simulink model "RC_Logitech"  (R2017b)
settings: Solver=FixedStepDiscrete  StartTime=0.0  StopTime=inf  FixedStep=0.02  RelTol=1e-3
libraries: simulink x16, aerolibanimutils x1
settings Model: Creator=juju  LastModifiedBy=zht
settings DataIOCC: LimitDataPoints=on  SaveFormat=Array  SaveOutput=off
settings OptimizationCC: BlockReduction=off  BooleanDataType=off  LifeSpan=inf
settings DebuggingCC: ConsistencyChecking=error  SignalInfNanChecking=error  SignalRangeChecking=error  ReadBeforeWriteMsg=EnableAllAsError  WriteAfterWriteMsg=EnableAllAsError  WriteAfterReadMsg=EnableAllAsError  AlgebraicLoopMsg=error  ArtificialAlgebraicLoopMsg=error  SaveWithDisabledLinksMsg=error  SaveWithParameterizedLinksMsg=error  BlockPriorityViolationMsg=error  MinStepSizeMsg=error  TimeAdjustmentMsg=warning  SolverPrmCheckMsg=error  InheritedTsInSrcMsg=error  SingleTaskRateTransMsg=error  TasksWithSamePriorityMsg=error  SigSpecEnsureSampleTimeMsg=error  CheckMatrixSingularityMsg=error  IntegerOverflowMsg=error  ParameterUnderflowMsg=error  ParameterPrecisionLossMsg=error  ParameterTunabilityLossMsg=error  FixptConstUnderflowMsg=error  FixptConstOverflowMsg=error  FixptConstPrecisionLossMsg=error  UnderSpecifiedDataTypeMsg=warning  UnnecessaryDatatypeConvMsg=warning  VectorMatrixConversionMsg=error  SignalLabelMismatchMsg=error  UnconnectedInputMsg=error  UnconnectedOutputMsg=error  UnconnectedLineMsg=error  SFcnCompatibilityMsg=error  UniqueDataStoreMsg=error  BusObjectLabelMismatch=error  RootOutportRequireBusObject=error  ModelReferenceIOMsg=error  ModelReferenceVersionMismatchMessage=error  ModelReferenceIOMismatchMessage=error  UnknownTsInhSupMsg=error  ModelReferenceDataLoggingMessage=error  StateNameClashWarn=warning  SimStateInterfaceChecksumMismatchMsg=error  StrictBusMsg=ErrorOnBusTreatedAsVector  BusNameAdapt=ErrorWithoutRepair  NonBusSignalsTreatedAsBus=error  SFUnusedDataAndEventsDiag=error  SFInvalidInputDataAccessInChartInitDiag=error  SFTransitionOutsideNaturalParentDiag=error  SFUnreachableExecutionPathDiag=error  SFUndirectedBroadcastEventsDiag=error  SFTransitionActionBeforeConditionDiag=error  SFTemporalDelaySmallerThanSampleTimeDiag=error  SFSelfTransitionDiag=error  SFExecutionAtInitializationDiag=error  SFMachineParentedDataDiag=error  IntegerSaturationMsg=error
settings HardwareCC: ProdBitPerPointer=32  ProdBitPerSizeT=32  ProdBitPerPtrDiffT=32  ProdLargestAtomicFloat=None  ProdIntDivRoundTo=Undefined  ProdEndianess=Unspecified  ProdWordSize=32  ProdHWDeviceType=32-bit Generic  TargetBitPerLong=64  TargetBitPerPointer=64  TargetBitPerSizeT=64  TargetBitPerPtrDiffT=64  TargetLongLongMode=on  TargetIntDivRoundTo=Zero  TargetEndianess=LittleEndian  TargetWordSize=64  TargetHWDeviceType=MATLAB Host  ProdEqTarget=off
settings ModelReferenceCC: PropagateSignalLabelsOutOfModel=off
settings CodeAppCC: StateflowObjectComments=on
settings GRTTargetCC: TargetLangStandard=C89/C90 (ANSI)  GeneratePreprocessorConditionals=Disable all
settings ConfigComp: CovMetricSettings=dw  CovHtmlReporting=on  CovSaveCumulativeToWorkspaceVar=on  CovSaveSingleToWorkspaceVar=on  CovExternalEMLEnable=off  CovSFcnEnable=off
settings SimscapeCC: SimscapeNormalizeSystem=off

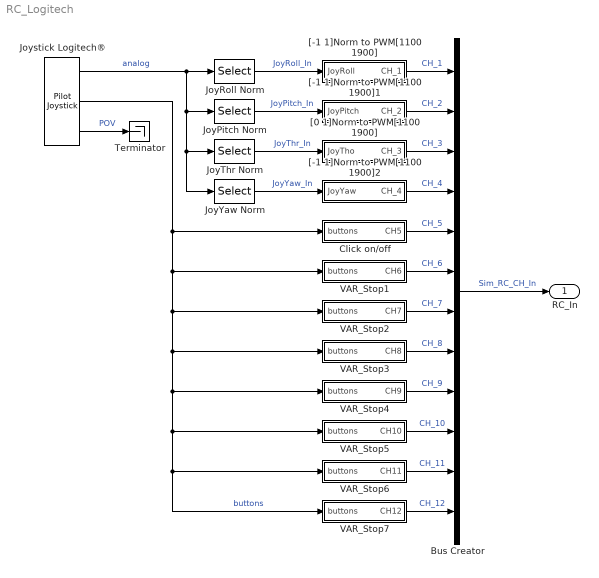
== system RC_Logitech ==
  Bus Creator : BusCreator  Inputs=12  OutDataTypeStr=Bus: RC_In_BUS  NonVirtualBus=on
  Click on/off : Subsystem
  JoyPitch Norm : Selector  InputPortWidth=6  IndexOptions=Index vector (dialog)  Indices=[2]  OutputSizes=1
  JoyRoll Norm : Selector  InputPortWidth=6  IndexOptions=Index vector (dialog)  Indices=[1]  OutputSizes=1
  JoyThr Norm : Selector  InputPortWidth=6  IndexOptions=Index vector (dialog)  Indices=[3]  OutputSizes=1
  JoyYaw Norm : Selector  InputPortWidth=6  IndexOptions=Index vector (dialog)  Indices=[4]  OutputSizes=1
  Joystick Logitech® : aerolibanimutils/Pilot Joystick  JoystickID=None  OutputConfiguration=AllOutputs  SampleTime=0.02
  Terminator : Terminator
  VAR_Stop1 : Subsystem
  VAR_Stop2 : Subsystem
  VAR_Stop3 : Subsystem
  VAR_Stop4 : Subsystem
  VAR_Stop5 : Subsystem
  VAR_Stop6 : Subsystem
  VAR_Stop7 : Subsystem
  "[-1 1]Norm to PWM[1100 1900]" : Subsystem
  "[-1 1]Norm to PWM[1100 1900]1" : Subsystem
  "[-1 1]Norm to PWM[1100 1900]2" : Subsystem
  "[0 1]Norm to PWM[1100 1900]" : Subsystem
  RC_In : Outport  OutDataTypeStr=Bus: RC_In_BUS
  wires:
  Joystick Logitech®/2 -> Click on/off/1(buttons), VAR_Stop1/1(buttons), VAR_Stop2/1(buttons), VAR_Stop3/1(buttons), VAR_Stop4/1(buttons), VAR_Stop5/1(buttons), VAR_Stop6/1(buttons), VAR_Stop7/1(buttons)  "buttons"
  Joystick Logitech®/3 -> Terminator/1  "POV"
  "[-1 1]Norm to PWM[1100 1900]"/1(CH_1) -> Bus Creator/1  "CH_1"
  "[-1 1]Norm to PWM[1100 1900]1"/1(CH_2) -> Bus Creator/2  "CH_2"
  "[0 1]Norm to PWM[1100 1900]"/1(CH_3) -> Bus Creator/3  "CH_3"
  "[-1 1]Norm to PWM[1100 1900]2"/1(CH_4) -> Bus Creator/4  "CH_4"
  Click on/off/1(CH5) -> Bus Creator/5  "CH_5"
  VAR_Stop1/1(CH6) -> Bus Creator/6  "CH_6"
  VAR_Stop2/1(CH7) -> Bus Creator/7  "CH_7"
  VAR_Stop3/1(CH8) -> Bus Creator/8  "CH_8"
  VAR_Stop5/1(CH10) -> Bus Creator/10  "CH_10"
  VAR_Stop4/1(CH9) -> Bus Creator/9  "CH_9"
  VAR_Stop6/1(CH11) -> Bus Creator/11  "CH_11"
  VAR_Stop7/1(CH12) -> Bus Creator/12  "CH_12"
  Joystick Logitech®/1 -> JoyYaw Norm/1, JoyThr Norm/1, JoyPitch Norm/1, JoyRoll Norm/1  "analog"
  JoyRoll Norm/1 -> "[-1 1]Norm to PWM[1100 1900]"/1(JoyRoll)  "JoyRoll_In"
  JoyPitch Norm/1 -> "[-1 1]Norm to PWM[1100 1900]1"/1(JoyPitch)  "JoyPitch_In"
  JoyThr Norm/1 -> "[0 1]Norm to PWM[1100 1900]"/1(JoyTho)  "JoyThr_In"
  JoyYaw Norm/1 -> "[-1 1]Norm to PWM[1100 1900]2"/1(JoyYaw)  "JoyYaw_In"
  Bus Creator/1 -> RC_In/1  "Sim_RC_CH_In"

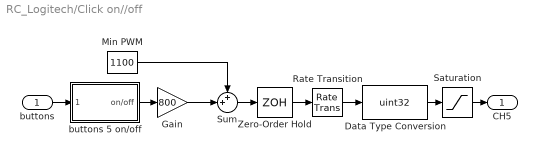
== system RC_Logitech/Click on//off ==
  buttons : Inport
  Data Type Conversion : DataTypeConversion  OutDataTypeStr=uint32
  Gain : Gain  Gain=800
  Min PWM : Constant  Value=1100
  Rate Transition : RateTransition
  Saturation : Saturate  UpperLimit=1900  LowerLimit=1100
  Sum : Sum  Inputs=++|
  Zero-Order Hold : ZeroOrderHold  SampleTime=0.02
  buttons 5 on/off : Subsystem
  CH5 : Outport
  wires:
  buttons/1 -> buttons 5 on/off/1(buttons)
  Min PWM/1 -> Sum/1
  Rate Transition/1 -> Data Type Conversion/1
  buttons 5 on/off/1(on/off) -> Gain/1
  Gain/1 -> Sum/2
  Data Type Conversion/1 -> Saturation/1
  Sum/1 -> Zero-Order Hold/1
  Zero-Order Hold/1 -> Rate Transition/1
  Saturation/1 -> CH5/1

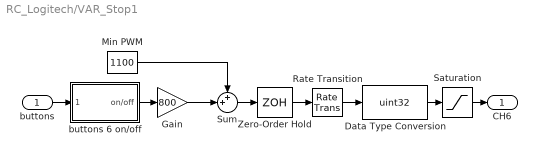
== system RC_Logitech/VAR_Stop1 ==
  buttons : Inport
  Data Type Conversion : DataTypeConversion  OutDataTypeStr=uint32
  Gain : Gain  Gain=800
  Min PWM : Constant  Value=1100
  Rate Transition : RateTransition
  Saturation : Saturate  UpperLimit=1900  LowerLimit=1100
  Sum : Sum  Inputs=++|
  Zero-Order Hold : ZeroOrderHold  SampleTime=0.02
  buttons 6 on/off : Subsystem
  CH6 : Outport
  wires:
  Saturation/1 -> CH6/1
  Zero-Order Hold/1 -> Rate Transition/1
  Sum/1 -> Zero-Order Hold/1
  Data Type Conversion/1 -> Saturation/1
  Gain/1 -> Sum/2
  buttons 6 on/off/1(on/off) -> Gain/1
  Rate Transition/1 -> Data Type Conversion/1
  Min PWM/1 -> Sum/1
  buttons/1 -> buttons 6 on/off/1(buttons)

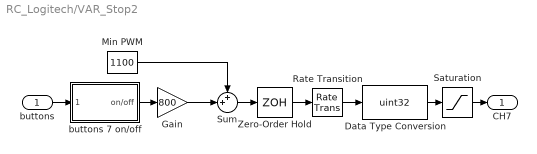
== system RC_Logitech/VAR_Stop2 ==
  buttons : Inport
  Data Type Conversion : DataTypeConversion  OutDataTypeStr=uint32
  Gain : Gain  Gain=800
  Min PWM : Constant  Value=1100
  Rate Transition : RateTransition
  Saturation : Saturate  UpperLimit=1900  LowerLimit=1100
  Sum : Sum  Inputs=++|
  Zero-Order Hold : ZeroOrderHold  SampleTime=0.02
  buttons 7 on/off : Subsystem
  CH7 : Outport
  wires:
  buttons/1 -> buttons 7 on/off/1(buttons)
  Min PWM/1 -> Sum/1
  Rate Transition/1 -> Data Type Conversion/1
  buttons 7 on/off/1(on/off) -> Gain/1
  Gain/1 -> Sum/2
  Data Type Conversion/1 -> Saturation/1
  Sum/1 -> Zero-Order Hold/1
  Zero-Order Hold/1 -> Rate Transition/1
  Saturation/1 -> CH7/1

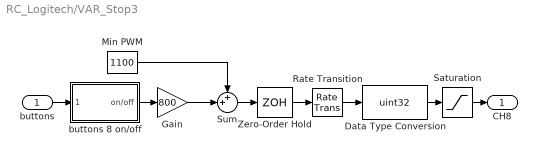
== system RC_Logitech/VAR_Stop3 ==
  buttons : Inport
  Data Type Conversion : DataTypeConversion  OutDataTypeStr=uint32
  Gain : Gain  Gain=800
  Min PWM : Constant  Value=1100
  Rate Transition : RateTransition
  Saturation : Saturate  UpperLimit=1900  LowerLimit=1100
  Sum : Sum  Inputs=++|
  Zero-Order Hold : ZeroOrderHold  SampleTime=0.02
  buttons 8 on/off : Subsystem
  CH8 : Outport
  wires:
  Saturation/1 -> CH8/1
  Zero-Order Hold/1 -> Rate Transition/1
  Sum/1 -> Zero-Order Hold/1
  Data Type Conversion/1 -> Saturation/1
  Gain/1 -> Sum/2
  buttons 8 on/off/1(on/off) -> Gain/1
  Rate Transition/1 -> Data Type Conversion/1
  Min PWM/1 -> Sum/1
  buttons/1 -> buttons 8 on/off/1(buttons)

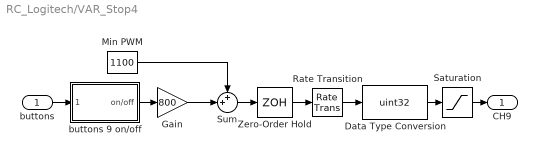
== system RC_Logitech/VAR_Stop4 ==
  buttons : Inport
  Data Type Conversion : DataTypeConversion  OutDataTypeStr=uint32
  Gain : Gain  Gain=800
  Min PWM : Constant  Value=1100
  Rate Transition : RateTransition
  Saturation : Saturate  UpperLimit=1900  LowerLimit=1100
  Sum : Sum  Inputs=++|
  Zero-Order Hold : ZeroOrderHold  SampleTime=0.02
  buttons 9 on/off : Subsystem
  CH9 : Outport
  wires:
  buttons/1 -> buttons 9 on/off/1(buttons)
  Min PWM/1 -> Sum/1
  Rate Transition/1 -> Data Type Conversion/1
  buttons 9 on/off/1(on/off) -> Gain/1
  Gain/1 -> Sum/2
  Data Type Conversion/1 -> Saturation/1
  Sum/1 -> Zero-Order Hold/1
  Zero-Order Hold/1 -> Rate Transition/1
  Saturation/1 -> CH9/1

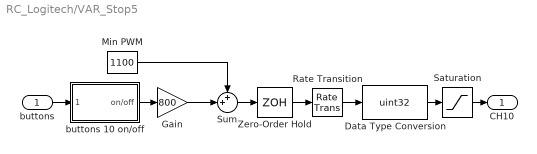
== system RC_Logitech/VAR_Stop5 ==
  buttons : Inport
  Data Type Conversion : DataTypeConversion  OutDataTypeStr=uint32
  Gain : Gain  Gain=800
  Min PWM : Constant  Value=1100
  Rate Transition : RateTransition
  Saturation : Saturate  UpperLimit=1900  LowerLimit=1100
  Sum : Sum  Inputs=++|
  Zero-Order Hold : ZeroOrderHold  SampleTime=0.02
  buttons 10 on/off : Subsystem
  CH10 : Outport
  wires:
  Saturation/1 -> CH10/1
  Zero-Order Hold/1 -> Rate Transition/1
  Sum/1 -> Zero-Order Hold/1
  Data Type Conversion/1 -> Saturation/1
  Gain/1 -> Sum/2
  buttons 10 on/off/1(on/off) -> Gain/1
  Rate Transition/1 -> Data Type Conversion/1
  Min PWM/1 -> Sum/1
  buttons/1 -> buttons 10 on/off/1(buttons)

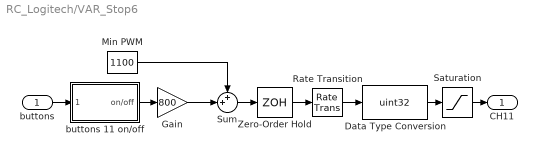
== system RC_Logitech/VAR_Stop6 ==
  buttons : Inport
  Data Type Conversion : DataTypeConversion  OutDataTypeStr=uint32
  Gain : Gain  Gain=800
  Min PWM : Constant  Value=1100
  Rate Transition : RateTransition
  Saturation : Saturate  UpperLimit=1900  LowerLimit=1100
  Sum : Sum  Inputs=++|
  Zero-Order Hold : ZeroOrderHold  SampleTime=0.02
  buttons 11 on/off : Subsystem
  CH11 : Outport
  wires:
  buttons/1 -> buttons 11 on/off/1(buttons)
  Min PWM/1 -> Sum/1
  Rate Transition/1 -> Data Type Conversion/1
  buttons 11 on/off/1(on/off) -> Gain/1
  Gain/1 -> Sum/2
  Data Type Conversion/1 -> Saturation/1
  Sum/1 -> Zero-Order Hold/1
  Zero-Order Hold/1 -> Rate Transition/1
  Saturation/1 -> CH11/1

== system RC_Logitech/VAR_Stop7 ==
  buttons : Inport
  Data Type Conversion : DataTypeConversion  OutDataTypeStr=uint32
  Gain : Gain  Gain=800
  Min PWM : Constant  Value=1100
  Rate Transition : RateTransition
  Saturation : Saturate  UpperLimit=1900  LowerLimit=1100
  Sum : Sum  Inputs=++|
  Zero-Order Hold : ZeroOrderHold  SampleTime=0.02
  buttons 12 on/off : Subsystem
  CH12 : Outport
  wires:
  Saturation/1 -> CH12/1
  Zero-Order Hold/1 -> Rate Transition/1
  Sum/1 -> Zero-Order Hold/1
  Data Type Conversion/1 -> Saturation/1
  Gain/1 -> Sum/2
  buttons 12 on/off/1(on/off) -> Gain/1
  Rate Transition/1 -> Data Type Conversion/1
  Min PWM/1 -> Sum/1
  buttons/1 -> buttons 12 on/off/1(buttons)

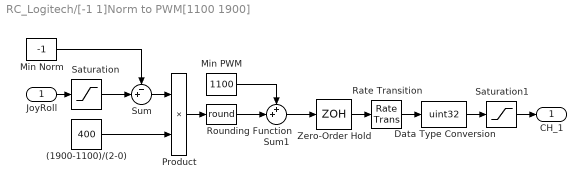
== system RC_Logitech/[-1 1]Norm to PWM[1100 1900] ==
  JoyRoll : Inport  OutDataTypeStr=double  Unit=1  PortDimensions=1
  (1900-1100)/(2-0) : Constant  Value=400  OutDataTypeStr=uint32
  Data Type Conversion : DataTypeConversion  OutDataTypeStr=uint32
  Min Norm : Constant  Value=-1
  Min PWM : Constant  Value=1100  OutDataTypeStr=uint32
  Product : Product  Inputs=**
  Rate Transition : RateTransition
  Rounding Function : Rounding  Operator=round
  Saturation : Saturate  UpperLimit=1  LowerLimit=-1
  Saturation1 : Saturate  UpperLimit=1900  LowerLimit=1100
  Sum : Sum  Inputs=-+|
  Sum1 : Sum  Inputs=++|
  Zero-Order Hold : ZeroOrderHold  SampleTime=0.02
  CH_1 : Outport  OutMin=[1100]  OutMax=[1900]  OutDataTypeStr=uint32  PortDimensions=1
  wires:
  JoyRoll/1 -> Saturation/1
  Saturation/1 -> Sum/2
  Min Norm/1 -> Sum/1
  Sum/1 -> Product/1
  (1900-1100)/(2-0)/1 -> Product/2
  Product/1 -> Rounding Function/1
  Min PWM/1 -> Sum1/1
  Sum1/1 -> Zero-Order Hold/1
  Rounding Function/1 -> Sum1/2
  Data Type Conversion/1 -> Saturation1/1
  Zero-Order Hold/1 -> Rate Transition/1
  Rate Transition/1 -> Data Type Conversion/1
  Saturation1/1 -> CH_1/1

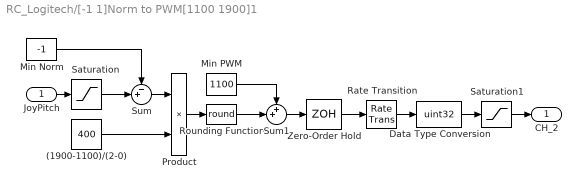
== system RC_Logitech/[-1 1]Norm to PWM[1100 1900]1 ==
  JoyPitch : Inport  OutDataTypeStr=double  Unit=1  PortDimensions=1
  (1900-1100)/(2-0) : Constant  Value=400
  Data Type Conversion : DataTypeConversion  OutDataTypeStr=uint32
  Min Norm : Constant  Value=-1
  Min PWM : Constant  Value=1100
  Product : Product  Inputs=**
  Rate Transition : RateTransition
  Rounding Function : Rounding  Operator=round
  Saturation : Saturate  UpperLimit=1  LowerLimit=-1
  Saturation1 : Saturate  UpperLimit=1900  LowerLimit=1100
  Sum : Sum  Inputs=-+|
  Sum1 : Sum  Inputs=++|
  Zero-Order Hold : ZeroOrderHold  SampleTime=0.02
  CH_2 : Outport  OutMin=[1100]  OutMax=[1900]  OutDataTypeStr=uint32  PortDimensions=1
  wires:
  Data Type Conversion/1 -> Saturation1/1
  Rounding Function/1 -> Sum1/2
  Min PWM/1 -> Sum1/1
  Product/1 -> Rounding Function/1
  (1900-1100)/(2-0)/1 -> Product/2
  Sum/1 -> Product/1
  Min Norm/1 -> Sum/1
  Saturation/1 -> Sum/2
  JoyPitch/1 -> Saturation/1
  Zero-Order Hold/1 -> Rate Transition/1
  Rate Transition/1 -> Data Type Conversion/1
  Saturation1/1 -> CH_2/1
  Sum1/1 -> Zero-Order Hold/1

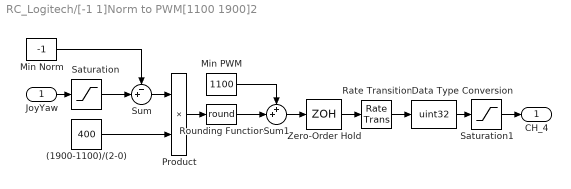
== system RC_Logitech/[-1 1]Norm to PWM[1100 1900]2 ==
  JoyYaw : Inport  OutDataTypeStr=double  Unit=1  PortDimensions=1
  (1900-1100)/(2-0) : Constant  Value=400
  Data Type Conversion : DataTypeConversion  OutDataTypeStr=uint32
  Min Norm : Constant  Value=-1
  Min PWM : Constant  Value=1100
  Product : Product  Inputs=**
  Rate Transition : RateTransition
  Rounding Function : Rounding  Operator=round
  Saturation : Saturate  UpperLimit=1  LowerLimit=-1
  Saturation1 : Saturate  UpperLimit=1900  LowerLimit=1100
  Sum : Sum  Inputs=-+|
  Sum1 : Sum  Inputs=++|
  Zero-Order Hold : ZeroOrderHold  SampleTime=0.02
  CH_4 : Outport  OutMin=[1100]  OutMax=[1900]  OutDataTypeStr=uint32  PortDimensions=1
  wires:
  JoyYaw/1 -> Saturation/1
  Saturation/1 -> Sum/2
  Min Norm/1 -> Sum/1
  Sum/1 -> Product/1
  (1900-1100)/(2-0)/1 -> Product/2
  Product/1 -> Rounding Function/1
  Min PWM/1 -> Sum1/1
  Sum1/1 -> Zero-Order Hold/1
  Rounding Function/1 -> Sum1/2
  Zero-Order Hold/1 -> Rate Transition/1
  Rate Transition/1 -> Data Type Conversion/1
  Data Type Conversion/1 -> Saturation1/1
  Saturation1/1 -> CH_4/1

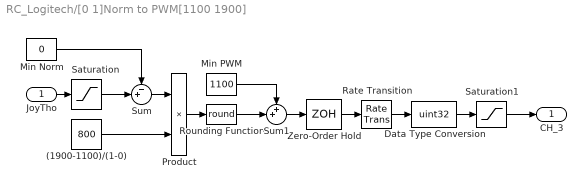
== system RC_Logitech/[0 1]Norm to PWM[1100 1900] ==
  JoyTho : Inport  OutDataTypeStr=double  Unit=1  PortDimensions=1
  (1900-1100)/(1-0) : Constant  Value=800
  Data Type Conversion : DataTypeConversion  OutDataTypeStr=uint32
  Min Norm : Constant  Value=0
  Min PWM : Constant  Value=1100
  Product : Product  Inputs=**
  Rate Transition : RateTransition
  Rounding Function : Rounding  Operator=round
  Saturation : Saturate  UpperLimit=1  LowerLimit=-1
  Saturation1 : Saturate  UpperLimit=1900  LowerLimit=1100
  Sum : Sum  Inputs=-+|
  Sum1 : Sum  Inputs=++|
  Zero-Order Hold : ZeroOrderHold  SampleTime=0.02
  CH_3 : Outport  OutMin=[1100]  OutMax=[1900]  OutDataTypeStr=uint32  PortDimensions=1
  wires:
  JoyTho/1 -> Saturation/1
  Saturation/1 -> Sum/2
  Min Norm/1 -> Sum/1
  Sum/1 -> Product/1
  (1900-1100)/(1-0)/1 -> Product/2
  Product/1 -> Rounding Function/1
  Min PWM/1 -> Sum1/1
  Rounding Function/1 -> Sum1/2
  Zero-Order Hold/1 -> Rate Transition/1
  Rate Transition/1 -> Data Type Conversion/1
  Data Type Conversion/1 -> Saturation1/1
  Sum1/1 -> Zero-Order Hold/1
  Saturation1/1 -> CH_3/1

== system RC_Logitech/Click on//off/buttons 5 on//off ==
  buttons : Inport
  ButtonOnOff : MATLAB Function  TreatAsAtomicUnit=on
  Compare To Constant : simulink/Logic and Bit Operations/Compare To Constant  relop===  const=1  OutDataTypeStr=boolean
  Data Type Conversion3 : DataTypeConversion  OutDataTypeStr=double
  Joystick button 5 : simulink/Logic and Bit Operations/Compare To Constant  relop===  const=16  OutDataTypeStr=boolean
  bts : Subsystem  TreatAsAtomicUnit=on
  on/off : Outport  OutDataTypeStr=boolean  PortDimensions=1
  wires:
  Data Type Conversion3/1 -> ButtonOnOff/1(bts)
  Compare To Constant/1 -> on/off/1
  Joystick button 5/1 -> bts/1(In1)
  buttons/1 -> Joystick button 5/1, bts/Trigger
  bts/1(Out1) -> Data Type Conversion3/1
  ButtonOnOff/1(led) -> Compare To Constant/1

== system RC_Logitech/VAR_Stop1/buttons 6 on//off ==
  buttons : Inport
  ButtonOnOff : MATLAB Function  TreatAsAtomicUnit=on
  Compare To Constant : simulink/Logic and Bit Operations/Compare To Constant  relop===  const=1  OutDataTypeStr=boolean
  Data Type Conversion3 : DataTypeConversion  OutDataTypeStr=double
  Joystick button : simulink/Logic and Bit Operations/Compare To Constant  relop===  const=32  OutDataTypeStr=boolean
  bts : Subsystem  TreatAsAtomicUnit=on
  on/off : Outport  OutDataTypeStr=boolean  PortDimensions=1
  wires:
  ButtonOnOff/1(led) -> Compare To Constant/1
  bts/1(Out1) -> Data Type Conversion3/1
  buttons/1 -> bts/Trigger, Joystick button/1
  Joystick button/1 -> bts/1(In1)
  Compare To Constant/1 -> on/off/1
  Data Type Conversion3/1 -> ButtonOnOff/1(bts)

== system RC_Logitech/VAR_Stop2/buttons 7 on//off ==
  buttons : Inport
  ButtonOnOff : MATLAB Function  TreatAsAtomicUnit=on
  Compare To Constant : simulink/Logic and Bit Operations/Compare To Constant  relop===  const=1  OutDataTypeStr=boolean
  Data Type Conversion3 : DataTypeConversion  OutDataTypeStr=double
  Joystick button : simulink/Logic and Bit Operations/Compare To Constant  relop===  const=64  OutDataTypeStr=boolean
  bts : Subsystem  TreatAsAtomicUnit=on
  on/off : Outport  OutDataTypeStr=boolean  PortDimensions=1
  wires:
  Data Type Conversion3/1 -> ButtonOnOff/1(bts)
  Compare To Constant/1 -> on/off/1
  Joystick button/1 -> bts/1(In1)
  buttons/1 -> Joystick button/1, bts/Trigger
  bts/1(Out1) -> Data Type Conversion3/1
  ButtonOnOff/1(led) -> Compare To Constant/1

== system RC_Logitech/VAR_Stop3/buttons 8 on//off ==
  buttons : Inport
  ButtonOnOff : MATLAB Function  TreatAsAtomicUnit=on
  Compare To Constant : simulink/Logic and Bit Operations/Compare To Constant  relop===  const=1  OutDataTypeStr=boolean
  Data Type Conversion3 : DataTypeConversion  OutDataTypeStr=double
  Joystick button : simulink/Logic and Bit Operations/Compare To Constant  relop===  const=128  OutDataTypeStr=boolean
  bts : Subsystem  TreatAsAtomicUnit=on
  on/off : Outport  OutDataTypeStr=boolean  PortDimensions=1
  wires:
  ButtonOnOff/1(led) -> Compare To Constant/1
  bts/1(Out1) -> Data Type Conversion3/1
  buttons/1 -> bts/Trigger, Joystick button/1
  Joystick button/1 -> bts/1(In1)
  Compare To Constant/1 -> on/off/1
  Data Type Conversion3/1 -> ButtonOnOff/1(bts)

== system RC_Logitech/VAR_Stop4/buttons 9 on//off ==
  buttons : Inport
  ButtonOnOff : MATLAB Function  TreatAsAtomicUnit=on
  Compare To Constant : simulink/Logic and Bit Operations/Compare To Constant  relop===  const=1  OutDataTypeStr=boolean
  Data Type Conversion3 : DataTypeConversion  OutDataTypeStr=double
  Joystick button : simulink/Logic and Bit Operations/Compare To Constant  relop===  const=256  OutDataTypeStr=boolean
  bts : Subsystem  TreatAsAtomicUnit=on
  on/off : Outport  OutDataTypeStr=boolean  PortDimensions=1
  wires:
  Data Type Conversion3/1 -> ButtonOnOff/1(bts)
  Compare To Constant/1 -> on/off/1
  Joystick button/1 -> bts/1(In1)
  buttons/1 -> Joystick button/1, bts/Trigger
  bts/1(Out1) -> Data Type Conversion3/1
  ButtonOnOff/1(led) -> Compare To Constant/1

== system RC_Logitech/VAR_Stop5/buttons 10 on//off ==
  buttons : Inport
  ButtonOnOff : MATLAB Function  TreatAsAtomicUnit=on
  Compare To Constant : simulink/Logic and Bit Operations/Compare To Constant  relop===  const=1  OutDataTypeStr=boolean
  Data Type Conversion3 : DataTypeConversion  OutDataTypeStr=double
  Joystick button : simulink/Logic and Bit Operations/Compare To Constant  relop===  const=512  OutDataTypeStr=boolean
  bts : Subsystem  TreatAsAtomicUnit=on
  on/off : Outport  OutDataTypeStr=boolean  PortDimensions=1
  wires:
  ButtonOnOff/1(led) -> Compare To Constant/1
  bts/1(Out1) -> Data Type Conversion3/1
  buttons/1 -> bts/Trigger, Joystick button/1
  Joystick button/1 -> bts/1(In1)
  Compare To Constant/1 -> on/off/1
  Data Type Conversion3/1 -> ButtonOnOff/1(bts)

== system RC_Logitech/VAR_Stop6/buttons 11 on//off ==
  buttons : Inport
  ButtonOnOff : MATLAB Function  TreatAsAtomicUnit=on
  Compare To Constant : simulink/Logic and Bit Operations/Compare To Constant  relop===  const=1  OutDataTypeStr=boolean
  Data Type Conversion3 : DataTypeConversion  OutDataTypeStr=double
  Joystick button : simulink/Logic and Bit Operations/Compare To Constant  relop===  const=1024  OutDataTypeStr=boolean
  bts : Subsystem  TreatAsAtomicUnit=on
  on/off : Outport  OutDataTypeStr=boolean  PortDimensions=1
  wires:
  Data Type Conversion3/1 -> ButtonOnOff/1(bts)
  Compare To Constant/1 -> on/off/1
  Joystick button/1 -> bts/1(In1)
  buttons/1 -> Joystick button/1, bts/Trigger
  bts/1(Out1) -> Data Type Conversion3/1
  ButtonOnOff/1(led) -> Compare To Constant/1

== system RC_Logitech/VAR_Stop7/buttons 12 on//off ==
  buttons : Inport
  ButtonOnOff : MATLAB Function  TreatAsAtomicUnit=on
  Compare To Constant : simulink/Logic and Bit Operations/Compare To Constant  relop===  const=1  OutDataTypeStr=boolean
  Data Type Conversion3 : DataTypeConversion  OutDataTypeStr=double
  Joystick button : simulink/Logic and Bit Operations/Compare To Constant  relop===  const=2048  OutDataTypeStr=boolean
  bts : Subsystem  TreatAsAtomicUnit=on
  on/off : Outport  OutDataTypeStr=boolean  PortDimensions=1
  wires:
  ButtonOnOff/1(led) -> Compare To Constant/1
  bts/1(Out1) -> Data Type Conversion3/1
  buttons/1 -> bts/Trigger, Joystick button/1
  Joystick button/1 -> bts/1(In1)
  Compare To Constant/1 -> on/off/1
  Data Type Conversion3/1 -> ButtonOnOff/1(bts)

== system RC_Logitech/Click on//off/buttons 5 on//off/bts ==
  In1 : Inport
  Trigger : TriggerPort  TriggerType=either  VariantControl=Variant  InitialTriggerSignalState=positive
  Out1 : Outport
  wires:
  In1/1 -> Out1/1

== system RC_Logitech/VAR_Stop1/buttons 6 on//off/bts ==
  In1 : Inport
  Trigger : TriggerPort  TriggerType=either  VariantControl=Variant  InitialTriggerSignalState=positive
  Out1 : Outport
  wires:
  In1/1 -> Out1/1

== system RC_Logitech/VAR_Stop2/buttons 7 on//off/bts ==
  In1 : Inport
  Trigger : TriggerPort  TriggerType=either  VariantControl=Variant  InitialTriggerSignalState=positive
  Out1 : Outport
  wires:
  In1/1 -> Out1/1

== system RC_Logitech/VAR_Stop3/buttons 8 on//off/bts ==
  In1 : Inport
  Trigger : TriggerPort  TriggerType=either  VariantControl=Variant  InitialTriggerSignalState=positive
  Out1 : Outport
  wires:
  In1/1 -> Out1/1

== system RC_Logitech/VAR_Stop4/buttons 9 on//off/bts ==
  In1 : Inport
  Trigger : TriggerPort  TriggerType=either  VariantControl=Variant  InitialTriggerSignalState=positive
  Out1 : Outport
  wires:
  In1/1 -> Out1/1

== system RC_Logitech/VAR_Stop5/buttons 10 on//off/bts ==
  In1 : Inport
  Trigger : TriggerPort  TriggerType=either  VariantControl=Variant  InitialTriggerSignalState=positive
  Out1 : Outport
  wires:
  In1/1 -> Out1/1

== system RC_Logitech/VAR_Stop6/buttons 11 on//off/bts ==
  In1 : Inport
  Trigger : TriggerPort  TriggerType=either  VariantControl=Variant  InitialTriggerSignalState=positive
  Out1 : Outport
  wires:
  In1/1 -> Out1/1

== system RC_Logitech/VAR_Stop7/buttons 12 on//off/bts ==
  In1 : Inport
  Trigger : TriggerPort  TriggerType=either  VariantControl=Variant  InitialTriggerSignalState=positive
  Out1 : Outport
  wires:
  In1/1 -> Out1/1

== matlab function RC_Logitech/VAR_Stop1/buttons 6 on//off/ButtonOnOff ==
  data: bts input; led output
function led = ButtonOnOff(bts)

persistent btsb                                                            % Initialization(To initialize a variable in embedded function) 
if isempty(btsb)
    btsb = 0;
end

persistent leds
if isempty(leds)
    leds = 0;
end

if ((bts~=btsb) && (bts ==1))                                              % bts is the button on or off in this time step 
    if (leds == 0)
        leds = 1;
    else
        leds = 0;
    end
    btsb = bts;                                                            % btsb is the button on or of in before time step    
end

if ((bts~=btsb) && (bts ==0))
    btsb = bts;
end
led = leds;                                                                % led on or off
%  end

== matlab function RC_Logitech/Click on//off/buttons 5 on//off/ButtonOnOff ==
  data: bts input; led output
function led = ButtonOnOff(bts)

persistent btsb                                                            % Initialization(To initialize a variable in embedded function) 
if isempty(btsb)
    btsb = 0;
end

persistent leds
if isempty(leds)
    leds = 0;
end

if ((bts~=btsb) && (bts ==1))                                              % bts is the button on or off in this time step 
    if (leds == 0)
        leds = 1;
    else
        leds = 0;
    end
    btsb = bts;                                                            % btsb is the button on or of in before time step    
end

if ((bts~=btsb) && (bts ==0))
    btsb = bts;
end
led = leds;                                                                % led on or off
%  end

== matlab function RC_Logitech/VAR_Stop2/buttons 7 on//off/ButtonOnOff ==
  data: bts input; led output
function led = ButtonOnOff(bts)

persistent btsb                                                            % Initialization(To initialize a variable in embedded function) 
if isempty(btsb)
    btsb = 0;
end

persistent leds
if isempty(leds)
    leds = 0;
end

if ((bts~=btsb) && (bts ==1))                                              % bts is the button on or off in this time step 
    if (leds == 0)
        leds = 1;
    else
        leds = 0;
    end
    btsb = bts;                                                            % btsb is the button on or of in before time step    
end

if ((bts~=btsb) && (bts ==0))
    btsb = bts;
end
led = leds;                                                                % led on or off
%  end

== matlab function RC_Logitech/VAR_Stop3/buttons 8 on//off/ButtonOnOff ==
  data: bts input; led output
function led = ButtonOnOff(bts)

persistent btsb                                                            % Initialization(To initialize a variable in embedded function) 
if isempty(btsb)
    btsb = 0;
end

persistent leds
if isempty(leds)
    leds = 0;
end

if ((bts~=btsb) && (bts ==1))                                              % bts is the button on or off in this time step 
    if (leds == 0)
        leds = 1;
    else
        leds = 0;
    end
    btsb = bts;                                                            % btsb is the button on or of in before time step    
end

if ((bts~=btsb) && (bts ==0))
    btsb = bts;
end
led = leds;                                                                % led on or off
%  end

== matlab function RC_Logitech/VAR_Stop4/buttons 9 on//off/ButtonOnOff ==
  data: bts input; led output
function led = ButtonOnOff(bts)

persistent btsb                                                            % Initialization(To initialize a variable in embedded function) 
if isempty(btsb)
    btsb = 0;
end

persistent leds
if isempty(leds)
    leds = 0;
end

if ((bts~=btsb) && (bts ==1))                                              % bts is the button on or off in this time step 
    if (leds == 0)
        leds = 1;
    else
        leds = 0;
    end
    btsb = bts;                                                            % btsb is the button on or of in before time step    
end

if ((bts~=btsb) && (bts ==0))
    btsb = bts;
end
led = leds;                                                                % led on or off
%  end

== matlab function RC_Logitech/VAR_Stop5/buttons 10 on//off/ButtonOnOff ==
  data: bts input; led output
function led = ButtonOnOff(bts)

persistent btsb                                                            % Initialization(To initialize a variable in embedded function) 
if isempty(btsb)
    btsb = 0;
end

persistent leds
if isempty(leds)
    leds = 0;
end

if ((bts~=btsb) && (bts ==1))                                              % bts is the button on or off in this time step 
    if (leds == 0)
        leds = 1;
    else
        leds = 0;
    end
    btsb = bts;                                                            % btsb is the button on or of in before time step    
end

if ((bts~=btsb) && (bts ==0))
    btsb = bts;
end
led = leds;                                                                % led on or off
%  end

== matlab function RC_Logitech/VAR_Stop6/buttons 11 on//off/ButtonOnOff ==
  data: bts input; led output
function led = ButtonOnOff(bts)

persistent btsb                                                            % Initialization(To initialize a variable in embedded function) 
if isempty(btsb)
    btsb = 0;
end

persistent leds
if isempty(leds)
    leds = 0;
end

if ((bts~=btsb) && (bts ==1))                                              % bts is the button on or off in this time step 
    if (leds == 0)
        leds = 1;
    else
        leds = 0;
    end
    btsb = bts;                                                            % btsb is the button on or of in before time step    
end

if ((bts~=btsb) && (bts ==0))
    btsb = bts;
end
led = leds;                                                                % led on or off
%  end

== matlab function RC_Logitech/VAR_Stop7/buttons 12 on//off/ButtonOnOff ==
  data: bts input; led output
function led = ButtonOnOff(bts)

persistent btsb                                                            % Initialization(To initialize a variable in embedded function) 
if isempty(btsb)
    btsb = 0;
end

persistent leds
if isempty(leds)
    leds = 0;
end

if ((bts~=btsb) && (bts ==1))                                              % bts is the button on or off in this time step 
    if (leds == 0)
        leds = 1;
    else
        leds = 0;
    end
    btsb = bts;                                                            % btsb is the button on or of in before time step    
end

if ((bts~=btsb) && (bts ==0))
    btsb = bts;
end
led = leds;                                                                % led on or off
%  end
